simulink model "pwm_test"  (R2015b)
settings: Solver=VariableStepAuto  StartTime=0.0  StopTime=9.4  RelTol=1e-3
undefined symbols (not defined in the file or in its folder): square, voltage_from_current, voltage_from_current1, voltage_from_current2
libraries: simulink x1
settings Model: Creator=sat_lab  LastModifiedBy=sat_lab

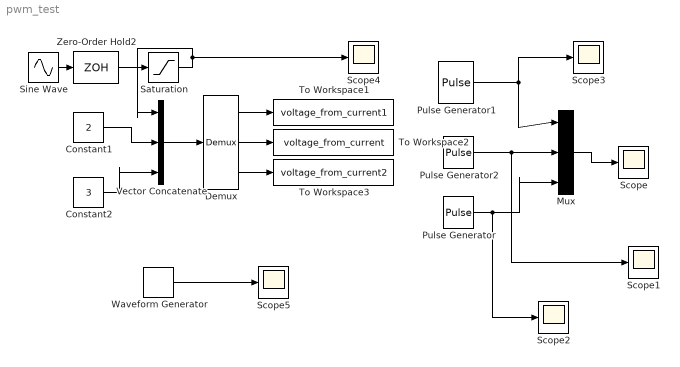
== system pwm_test ==
  Constant1 : Constant  Value=2
  Constant2 : Constant  Value=3
  Demux : Demux  Outputs=3
  Mux : Mux  Inputs=3
  Pulse Generator : DiscretePulseGenerator  PulseType=Time based  Amplitude=3.6  Period=1/5  PulseWidth=voltage_from_current2*100/3.6
  Pulse Generator1 : DiscretePulseGenerator  PulseType=Time based  Amplitude=3.6  Period=1/5  PulseWidth=voltage_from_current1*100/3.6
  Pulse Generator2 : DiscretePulseGenerator  PulseType=Time based  Amplitude=3.6  Period=1/5  PulseWidth=voltage_from_current*100/3.6
  Saturation : Saturate  UpperLimit=inf  LowerLimit=0.0001
  Scope{,1..5} (6 alike) : Scope
  Sine Wave : Sin  Amplitude=2  Frequency=2*pi  SampleTime=0
  To Workspace1 : ToWorkspace  VariableName=voltage_from_current1  SampleTime=-1
      settings: MaxDataPoints=1
  To Workspace2 : ToWorkspace  VariableName=voltage_from_current  SampleTime=-1
      settings: MaxDataPoints=1
  To Workspace3 : ToWorkspace  VariableName=voltage_from_current2  SampleTime=-1
      settings: MaxDataPoints=1
  Vector Concatenate : Concatenate  NumInputs=3
  Waveform Generator : simulink/Sources/Waveform Generator  OutMin=[]  OutMax=[]  OutDataTypeStr=double  SelectedSignal=1  Signals=square('Amplitude',3.6,'Frequency',5,'DutyCycle',voltage_from_current1*100/3.6)  BlockNames=MultiportSwitch_e7335084f7b14b1  SampleTime=.1
  Zero-Order Hold2 : ZeroOrderHold  SampleTime=0.25
  wires:
  Constant1/1 -> Vector Concatenate/2
  Constant2/1 -> Vector Concatenate/3
  Vector Concatenate/1 -> Demux/1
  Demux/1 -> To Workspace1/1
  Demux/2 -> To Workspace2/1
  Demux/3 -> To Workspace3/1
  Pulse Generator1/1 -> Mux/1, Scope3/1
  Pulse Generator2/1 -> Scope1/1, Mux/2
  Pulse Generator/1 -> Scope2/1, Mux/3
  Mux/1 -> Scope/1
  Sine Wave/1 -> Zero-Order Hold2/1
  Zero-Order Hold2/1 -> Saturation/1
  Saturation/1 -> Vector Concatenate/1, Scope4/1
  Waveform Generator/1 -> Scope5/1
